simulink model "LateralControllerDIY"  (R2021a)
settings: Solver=VariableStepAuto  StartTime=0.0  StopTime=20  RelTol=1e-3
values from neighbouring files (symbols this model uses):
  ks = 0    [controller_setup.m]    (also in test.m)
  PredictionHorizon = 60    [controller_setup.m]
  Ts = 0.05    [controller_setup.m]    (also in test.m = 0.1)
  Vx = 15    [controller_setup.m]    (also in test.m)
libraries: simulink_extras x3, mpclib x1
(part 2 of 2)

== matlab function LateralControllerDIY/MATLAB Function1 ==
  data: Vyr input; U1_out output; Yawr input; Rater input; Yr input; Fyr input; Mxr input; Vyc input; Yawc input; Ratec input; Yc input; Ulast1 input; Ulast2 input; Vx input; ks input; Useq input; U2_out output; Useq_ output; fval output; exitflag output; delta_t output; emax input; emin input
function [U1_out,U2_out,Useq_,fval,exitflag,delta_t] = fcn(Vyr,Yawr,Rater,Yr, Fyr,Mxr,Vyc,Yawc,Ratec,Yc,Ulast1,Ulast2,Vx,ks,Useq,emax,emin)
%Vyr lateral velocity, Yawr yaw angle, Rater yaw rate, Yr lateral position
%Fyr lateral force in front tyre,Mxr moment generated by longitudinal force
%'r'means reference ||  'c'means current
% Ulast1,Ulast2 are u(k-1), Ucrnt1,Ucrnt2 are u(k) calculated from last
% control period
    if Vx<0.1
        Vx=0.001;%make sure many expressions' denominator isn't 0
    end
    lr=1.67;%distance from mass center to rear axle
    threshold=0.1022;%critical slip angle before saturation
    miu=0.7;%friction coeficient
    rmax=9.81*miu/Vx;
%% Initilization    
    tstart=tic;%timing on
    
    Nx=4;%number of state
    Nu=2;%number of control(FOH should be twice)
    Np=70;%prediction horizon
    %N1 cannot be equal to N2
    N1=40;
    N2=10;
%     N3=20;
    Nc=1;%control horizon

    %reference
    r=zeros(Nx,1);%state reference
    r(1)=Vyr;
    r(2)=Yawr;
    r(3)=Rater;
    r(4)=Yr;    
    ur1=Fyr;
    ur2=Mxr;%control reference
    
    %states
    x=zeros(Nx,1);%state reference
    x(1)=Vyc;
    x(2)=Yawc;
    x(3)=Ratec;
    x(4)=Yc;   
    
    %control
    u=zeros(Nu,1);%state reference
    u(1)=Ulast1;
    u(2)=Ulast2;
    
    %get augmented states
    kesi=zeros(Nx+Nu,1);%[X;U]
    kesi(1)=x(1)-r(1);
    kesi(2)=x(2)-r(2);
    kesi(3)=x(3)-r(3);
    kesi(4)=x(4)-r(4);
    kesi(5)=u(1)-ur1;
    kesi(6)=u(2)-ur2;
    
%% Modellng->Discretization->prediction->quadratic programming
    %sample time 
    Ts1=0.01;%short sample time
    Ts2=0.2; %long sample time
    %Modelling&Linearization&Discretization
    steps=Np+1;
    A = zeros(Nx+Nu,Nx+Nu,steps);
    B = zeros(Nx+Nu,Nu*2,steps);
    Dc = zeros(Nx+Nu,1,steps);
    C=[1 0 0 0 0 0;0 1 0 0 0 0;0 0 1 0 0 0;0 0 0 1 0 0];
    
    for ct = 1:steps
        uk = Useq(ct,:);
        if ct == steps
            uk1 = Useq(ct,:);
        else
            uk1= Useq(ct+1,:);
        end
        uk=uk';
        uk1=uk1';
        if ct<=N1 %in short prediction region, using zero order hold
            Ts=Ts1;
            [Ad, Bd, DK, delta_x] = GetDynamicsZOH(Vx,ks,x,uk,Ts);
            A(:,:,ct)=[Ad,Bd;zeros(Nu,Nx),eye(Nu)];        
            B(:,:,ct)=[Bd zeros(4,2);eye(Nu) zeros(2,2)];%in order to fit the dimension of B from ZOH with B from FOH, augumentation is done here
            Dc(:,:,ct)=[DK;0;0];%constant component
        elseif ct<=N1+N2 %in correction prediction region, using first order hold
            Ts=Ts1+(Ts2-Ts1)*(ct-N1)/(N2-N1);%get this step's correction sample time
            [Ad, Bd1,Bd2, DK, delta_x] = GetDynamicsFOH(Vx,ks,x,uk,uk1,Ts);
            A(:,:,ct)=[Ad Bd1+Bd2;zeros(Nu,Nx) eye(Nu)];        
            B(:,:,ct)=[Bd1+Bd2 Bd2;eye(Nu) zeros(Nu,Nu)];
            Dc(:,:,ct)=[DK;0;0];
        else %in long prediction region, using first order hold
            Ts=Ts2;
            [Ad, Bd1,Bd2, DK, delta_x] = GetDynamicsFOH(Vx,ks,x,uk,uk1,Ts);
            A(:,:,ct)=[Ad Bd1+Bd2;zeros(Nu,Nx) eye(Nu)];        
            B(:,:,ct)=[Bd1+Bd2 Bd2;eye(Nu) zeros(Nu,Nu)];
            Dc(:,:,ct)=[DK;0;0];
        end    
        x=x+delta_x;    %predict next step's states
    end
    %construct important matrix
    %Y=PHI*kesi+THETA*delta_U+OMEGA*D
    coder.varsize('PHI',[Np*Nx,Nx+Nu]);
    coder.varsize('THETA',[Np*Nx,2*Nu]);
    coder.varsize('D',[Np*(Nx+Nu),1]);
    coder.varsize('DD',[Np*Nx,1]);
    PHI=[];
    THETA=zeros(Np*Nx,2*Nu);
    D=[];
    product=eye(6);
    for j=1:Np
        product=A(:,:,j)*product;
        PHI=[PHI;C*product];
        D=[D;Dc(:,:,j)];
    end
    for k=1:Nc
        product1=eye(6);
        for j=k:Np
            THETA(4*j-3:4*j,4*k-3:4*k)=C*product1*B(:,:,Nc);
            product1=A(:,:,j+1)*product1;
        end
    end
    coder.varsize('OMEGA',[Nx*Np,(Nx+Nu)*Np]);
    OMEGA=zeros(Nx*Np,(Nx+Nu)*Np);
    for i=1:Np
        product2=A(:,:,i+1);
        for j=i:Np-1
            if i==j
                OMEGA(4*i-3:4*i,6*i-5:6*i)=C*eye(6);
            end
            OMEGA(4*j+1:4*j+4,6*j+1:6*j+6)=C*product2;
            product2=A(:,:,j+2)*product2;
        end
    end
    DD=OMEGA*D;        
    Sigma=repmat([1 0 1 0;0 1 0 1],Np,1);
    Sigma(1:2,1:4)=[1 0 0 0;0 1 0 0];%in cost function: (UT+Sigma*deltaU)'*R*(UT+Sigma*deltaU)
    UT=kron(ones(Np,1),[u(1);u(2)]); %=repmat([u(1);u(2);u(3);u(4)],Np,1) %(Nu*Np,1)
    error=PHI*kesi;%(Nx*Np,Nx+Nu)*(Nu+Nx,1)
    Q=kron(eye(Np,Np),diag([0 0 100 4])); %weight matrix for output  
    R=kron(eye(Np,Np),diag([0 4e-5]));    %weight matrix for control  
    P=diag([3e-5 8e-5 3e-5 8e-5]);        %weight matrix for control increment (???P=diag([3e-5 8e-5 3e-5 8e-5]) or diag([3e-5 8e-5 0 0])  )
    rou1=3e3;                             %weight for handling envelop slack variable
    rou2=5e6;                             %weight for enviroment envelop slack variable(it is 5e4 in the paper)
    H=2*[THETA'*Q*THETA+Sigma'*R*Sigma+P zeros(4,2);zeros(1,4) rou1 0;zeros(1,4) 0 rou2];   %double check if it is mutiplied with 2
    f=[2*(error'*Q*THETA+(OMEGA*D)'*Q*THETA+UT'*R*Sigma),0,0];                              %seems transpose or not doesn't make a difference
   %% constraints
    %inequation
    A_I=[1 0 0 0;0 1 0 0;1 0 1 0;0 1 0 1];%[u(k),u(k+1),u(k+2)...u(k+Nc)]'=A_I*deltaU 
    Ut=kron(ones(2,1),[Ulast1;Ulast2]);%control in last control step
    umin=[-1e4; -1e3];
    umax=[1e4; 1e3];
    Umin=kron(ones(2,1),umin);  %lower boud for control
    Umax=kron(ones(2,1),umax);  %upper boud for control
    coder.varsize('A_cons',[Np*6+8,6]);
    coder.varsize('b_cons',[Np*6+8,1]);
    %bound for control
    A_cons=[A_I zeros(4,2);-A_I zeros(4,2)];  
    b_cons=[Umax-Ut;-Umin+Ut];
    %add constraints( handling envelop & environment envolop)
    gamas=[1 -lr 0 0;-1 lr 0 0;0 1 0 0;0 -1 0 0];
    gamae=[0 0 0 1;0 0 0 -1];
    Gs=[Vx*threshold;Vx*threshold;rmax;rmax];
    for i=1:Np
        A_cons=[A_cons;[gamas*THETA(4*i-3:4*i,:) -ones(4,1) zeros(4,1)];[gamae*THETA(4*i-3:4*i,:) zeros(2,1) -ones(2,1)]];
        b_cons=[b_cons;[Gs-gamas*(PHI(4*i-3:4*i,:)*kesi-DD(4*i-3:4*i,:))];[emax(i);-emin(i)]-gamae*(PHI(4*i-3:4*i,:)*kesi-DD(4*i-3:4*i,:))];
    end
    
    %upper and lower boundary
    delta_umin=[-1e4;-1e3]; %lower boud for control increment
    delta_umax=[1e4;1e3];   %upper boud for control increment
    M1=10;                  %upper bound handling envelop slack variable
    M2=10;                  %upper bound enviroment envelop slack variable
    delta_Umin=kron(ones(2,1),delta_umin);
    delta_Umax=kron(ones(2,1),delta_umax);
    lb=[delta_Umin;0;0];
    ub=[delta_Umax;M1;M2];  
   %% solve quadratic programming
    opts = optimoptions('quadprog','Algorithm','active-set');
    x_start=zeros(Nu*2+2,1);        %initial condition for DeltaU=[deltaU1,deltaU2,deltaU1next,deltaU2next,epsilon1,epsilon2]
    [X,fval,exitflag]=quadprog(H,f',A_cons,b_cons,[],[],lb,ub,x_start,opts);   %solve quadratic programmming
    
   %% calculate control signal
    U1=kesi(5)+X(1);%The output error at the previous time plus the optimization result to get the error at this time
    U2=kesi(6)+X(2);%The output error at the previous time plus the optimization result to get the error at this time
    U1_out=U1+ur1;%Error plus reference value to get final output value    
    U2_out=U2+ur2;
    Useq_=[U1_out U2_out; repmat([U1_out+X(3) U2_out+X(4)],Np,1)];
    delta_t=toc(tstart);%timing off
end

function [A, B, DK, delta_x] = GetDynamicsZOH(Vx,ks,x,u,Ts)
%Zero order hold discretization
%Plant Model parameters
m = 2272;   %mass
Iz = 4600;  %rotational inertia
lf = 1.11;  % distance from front axle to the mass center
lr = 1.67;  % distance from rear axle to the mass center
C_a = 1.822e5; % rear cornering stiffness 

%Enviroment parameters
miu = 0.7; %frction cooeficient 0.7 for dry road and 0.4 for wet
g = 9.81; % gravity

Fz = m*g*lf/(lf+lr); % the load that beared by the rear tire

%calculate alpha
Vy = x(1); %lateral velocity
r = x(2);  %yaw rate
alphar_ = Vy/Vx-lr*r/Vx;   %calculate linearzing point

%tire model
threshold = atan(3*miu*Fz/C_a);     % threshold for the tire linear region
if abs(alphar_)<threshold
    %the rear lateral force value (f(x0)) at the linearzing point
    Fyr_ = -C_a*tan(alphar_)+C_a^2/(3*miu*Fz)*abs(tan(alphar_))*tan(alphar_)-C_a^3/(27*miu^2*Fz^2)*tan(alphar_)^3;
    
    %the slope of linearized model (f‘(x0))
    if alphar_>= 0
        Cr_ = -C_a*sec(alphar_)^2+C_a^2/(3*miu*Fz)*(2*sec(alphar_)^2*tan(alphar_))-C_a^3/(27*miu^2*Fz^2)*(3*tan(alphar_)^2*sec(alphar_)^2);
    else
        Cr_ = -C_a*sec(alphar_)^2-C_a^2/(3*miu*Fz)*(2*sec(alphar_)^2*tan(alphar_))-C_a^3/(27*miu^2*Fz^2)*(3*tan(alphar_)^2*sec(alphar_)^2);
    end
else
    
    %the saturation region of tire model
    Fyr_ = -miu*Fz*sign(alphar_);
    Cr_ = 0;
end

%Continuous-time model
Ac = [Cr_/(m*Vx) -lr*Cr_/(m*Vx)-Vx 0 0;
    -lr*Cr_/(Iz*Vx) lr^2*Cr_/(Iz*Vx) 0 0;
    0 1 0 0;
    1 0 Vx 0];
Bc = [1/m 0;
    lf/Iz 1/Iz;
    0 0;
    0 0];
dcc = [(Fyr_-Cr_*alphar_)/m;
    -lr*(Fyr_-Cr_*alphar_)/Iz;
    -Vx*ks;
    0];

G=[Ac Bc dcc;zeros(3,7)];
M=expm(G*Ts);
A=M(1:4,1:4);
B=M(1:4,5:6);
DK=M(1:4,7);
delta_x=A*x+B*u+DK-x;
%%x(k+1)=A*x(k)+B*u(k)+DK
end

function [A, B1, B2, DK, delta_x] = GetDynamicsFOH(Vx,ks,x,uk,uk1,Ts)

%Plant Model parameters
m = 2272;   %mass
Iz = 4600;  %rotational inertia
lf = 1.11;  % distance from front axle to the mass center
lr = 1.67;  % distance from rear axle to the mass center
C_a = 1.822e5; % rear cornering stiffness 

%Enviroment parameters
miu = 0.7; %frction cooeficient 0.7 for dry road and 0.4 for wet
g = 9.81; % gravity

Fz = m*g*lf/(lf+lr); % the load that beared by the rear tire

%calculate alpha
Vy = x(1); %lateral velocity
r = x(2);  %yaw rate
alphar_ = Vy/Vx-lr*r/Vx;   %calculate linearzing point

%tire model
threshold = atan(3*miu*Fz/C_a);     % threshold for the tire linear region
if abs(alphar_)<threshold
    %the rear lateral force value (f(x0)) at the linearzing point
    Fyr_ = -C_a*tan(alphar_)+C_a^2/(3*miu*Fz)*abs(tan(alphar_))*tan(alphar_)-C_a^3/(27*miu^2*Fz^2)*tan(alphar_)^3;
    
    %the slope of linearized model (f‘(x0))
    if alphar_>= 0
        Cr_ = -C_a*sec(alphar_)^2+C_a^2/(3*miu*Fz)*(2*sec(alphar_)^2*tan(alphar_))-C_a^3/(27*miu^2*Fz^2)*(3*tan(alphar_)^2*sec(alphar_)^2);
    else
        Cr_ = -C_a*sec(alphar_)^2-C_a^2/(3*miu*Fz)*(2*sec(alphar_)^2*tan(alphar_))-C_a^3/(27*miu^2*Fz^2)*(3*tan(alphar_)^2*sec(alphar_)^2);
    end
else
    
    %the saturation region of tire model
    Fyr_ = -miu*Fz*sign(alphar_);
    Cr_ = 0;
end

%Continuous-time model
Ac = [Cr_/(m*Vx) -lr*Cr_/(m*Vx)-Vx 0 0;
    -lr*Cr_/(Iz*Vx) lr^2*Cr_/(Iz*Vx) 0 0;
    0 1 0 0;
    1 0 Vx 0];
Bc = [1/m 0;
    lf/Iz 1/Iz;
    0 0;
    0 0];
dcc = [(Fyr_-Cr_*alphar_)/m;
    -lr*(Fyr_-Cr_*alphar_)/Iz;
    -Vx*ks;
    0];

LAMDA=[Ac Bc dcc zeros(4,3);zeros(3,7) 1/Ts*eye(3);zeros(3,10)];
M=expm(LAMDA*Ts);
A=M(1:4,1:4);
PHI1=M(1:4,5:7);
PHI2=M(1:4,8:10);
B1=(PHI1-PHI2)*[eye(2);zeros(1,2)];
B2=PHI2*[eye(2);zeros(1,2)];
DK=PHI1*[0;0;1];
delta_x=A*x+B1*uk+B2*uk1+DK-x;
%%x(k+1)=A*x(k)+B1*u(k)=B2*u(k+1)+DK
end
